simulink model "Project"  (R2017a)
settings: Solver=VariableStepAuto  StartTime=0.0  StopTime=20  FixedStep=0.01  RelTol=1e-3
values from neighbouring files (symbols this model uses):
  b = 2    [initial_condition_and_plots.m]
  c = 4    [initial_condition_and_plots.m]
  C = 2    [initial_condition_and_plots.m]
  Dmax = 3    [initial_condition_and_plots.m]
  init1 = [ -29 -27 pi/6]    [initial_condition_and_plots.m]
  init2 = [ -27 -24 2*pi/3]    [initial_condition_and_plots.m]
  init3 = [ -25 -21 pi/12]    [initial_condition_and_plots.m]
  init4 = [ -23 -19 pi/2]    [initial_condition_and_plots.m]
  init5 = [ -21 -12 5*pi/4]    [initial_condition_and_plots.m]
  K = 4    [initial_condition_and_plots.m]
  K_th = 3    [initial_condition_and_plots.m]
  Kij = 3    [initial_condition_and_plots.m]
  L = 20    [initial_condition_and_plots.m]
  r1k = 3    [initial_condition_and_plots.m]
  r2k = 4    [initial_condition_and_plots.m]
  x1k = 0    [initial_condition_and_plots.m]
  x2k = 15    [initial_condition_and_plots.m]
  y1k = -20    [initial_condition_and_plots.m]
  y2k = -5    [initial_condition_and_plots.m]
  yd = @(i) 4*i-20    [initial_condition_and_plots.m]
(part 2 of 2)

== system Project/Robot 4/Tracking Control ==
  note: u(6) =th _d
  note: u(5) = error_th
  note: u(4) = derror_y
  note: u(3) = error_y
  note: u(2) = derror_x
  note: u(1) = error_x
  X1 : Inport
  Xd : Inport  Port=2
  Y1 : Inport  Port=3
  Yd : Inport  Port=4
  TH1 : Inport  Port=5
  THc : Inport  Port=6
  Dc : Inport  Port=7
  CC : Inport  Port=8
  CCD : InportShadow  Port=8
  CCTH : InportShadow  Port=8
  Constant : Constant  Value=Dmax
  Derivative2 : Derivative
  Derivative3 : Derivative
  Fcn : Fcn  Expr=K*cos( u(5) )*u(7)
  Fcn1 : Fcn  Expr=K * cos(u(5)) * sin( u(5) + u(6) )*u(7)
  Fcn2 : Fcn  Expr=-K_th*u(5) +u(8)*( u(1)*u(4) - u(3)*u(2) )/( u(1)^2+u(3)^2 )
  Fcn3 : Fcn  Expr=atan2(-u(1),-u(2))
  Fcn4 : Fcn  Expr=(u(1)^2+u(2)^2)*(1/2)
  Fcn5 : Fcn  Expr=cos(u(5)+u(6))
  Integrator1 : Integrator  InitialCondition=init4(2)
  Integrator2 : Integrator  InitialCondition=init4(3)
  Integrator3 : Integrator  InitialCondition=init4(1)
  MinMax : MinMax  Inputs=2
  Mux : Mux  Inputs=8
  Mux1 : Mux  Inputs=2
  Mux2 : Mux  Inputs=2
  Product : Product
  Scope : Scope
  Sum : Sum  Inputs=|-+
  Sum1 : Sum  Inputs=|-+
  Sum2 : Sum  Inputs=|+-
  Sum3 : Sum  Inputs=|+-
  Sum4 : Sum  Inputs=|+-
  Switch : Switch  Criteria=u2 ~= 0
  Switch1 : Switch  Criteria=u2 ~= 0
  Unit Delay : UnitDelay  SampleTime=-1
  Unit Delay1 : UnitDelay  SampleTime=-1
  X : Outport
  Y : Outport  Port=2
  "TH " : Outport  Port=3
  V : Outport  Port=4
  "U " : Outport  Port=5
  wires:
  Integrator1/1 -> Y/1
  Integrator3/1 -> X/1
  Fcn2/1 -> "U "/1, Integrator2/1
  Fcn1/1 -> Sum3/1, Integrator1/1
  Product/1 -> Sum4/1, Integrator3/1
  Fcn5/1 -> Product/2
  Fcn/1 -> Product/1, V/1
  Constant/1 -> MinMax/1
  Integrator2/1 -> "TH "/1
  Mux/1 -> Fcn5/1, Fcn/1, Fcn2/1, Fcn1/1
  Mux1/1 -> Fcn3/1
  Derivative2/1 -> Sum4/2
  Sum2/1 -> Mux/5
  Yd/1 -> [yd], Sum1/1
  Mux2/1 -> Fcn4/1
  [error_y] -> Mux2/2
  Sum/1 -> Mux/1, [error_x]
  [dy1] -> Unit Delay1/1
  [error_x] -> Mux2/1
  Sum3/1 -> [dy1]
  X1/1 -> Sum/2
  TH1/1 -> Sum2/1
  [error_y] -> Mux1/1
  [yd] -> Derivative3/1
  Sum4/1 -> [dx1]
  Derivative3/1 -> Sum3/2
  [error_x] -> Mux1/2
  Sum1/1 -> Mux/3, [error_y]
  Y1/1 -> Sum1/2
  [xd] -> Derivative2/1
  MinMax/1 -> Scope/1, Mux/7
  Xd/1 -> Sum/1, [xd]
  CC/1 -> Mux/8
  Fcn4/1 -> Switch/1
  Dc/1 -> Switch/3
  CCD/1 -> Switch/2
  Switch/1 -> MinMax/2
  Fcn3/1 -> Switch1/1
  THc/1 -> Switch1/3
  Switch1/1 -> Sum2/2, Mux/6
  CCTH/1 -> Switch1/2
  [dx1] -> Unit Delay/1
  Unit Delay/1 -> Mux/2
  Unit Delay1/1 -> Mux/4

== system Project/Robot 5/Tracking Control ==
  note: u(1) = error_x
  note: u(2) = derror_x
  note: u(3) = error_y
  note: u(4) = derror_y
  note: u(5) = error_th
  note: u(6) =th _d
  X1 : Inport
  Xd : Inport  Port=2
  Y1 : Inport  Port=3
  Yd : Inport  Port=4
  TH1 : Inport  Port=5
  THc : Inport  Port=6
  Dc : Inport  Port=7
  CC : Inport  Port=8
  CCD : InportShadow  Port=8
  CCTH : InportShadow  Port=8
  Constant : Constant  Value=Dmax
  Derivative2 : Derivative
  Derivative3 : Derivative
  Fcn : Fcn  Expr=K*cos( u(5) )*u(7)
  Fcn1 : Fcn  Expr=K * cos(u(5)) * sin( u(5) + u(6) )*u(7)
  Fcn2 : Fcn  Expr=-K_th*u(5) +u(8)*( u(1)*u(4) - u(3)*u(2) )/( u(1)^2+u(3)^2 )
  Fcn3 : Fcn  Expr=atan2(-u(1),-u(2))
  Fcn4 : Fcn  Expr=(u(1)^2+u(2)^2)*(1/2)
  Fcn5 : Fcn  Expr=cos(u(5)+u(6))
  Integrator1 : Integrator  InitialCondition=init5(2)
  Integrator2 : Integrator  InitialCondition=init5(3)
  Integrator3 : Integrator  InitialCondition=init5(1)
  MinMax : MinMax  Inputs=2
  Mux : Mux  Inputs=8
  Mux1 : Mux  Inputs=2
  Mux2 : Mux  Inputs=2
  Product : Product
  Scope : Scope
  Sum : Sum  Inputs=|-+
  Sum1 : Sum  Inputs=|-+
  Sum2 : Sum  Inputs=|+-
  Sum3 : Sum  Inputs=|+-
  Sum4 : Sum  Inputs=|+-
  Switch : Switch  Criteria=u2 ~= 0
  Switch1 : Switch  Criteria=u2 ~= 0
  Unit Delay : UnitDelay  SampleTime=-1
  Unit Delay1 : UnitDelay  SampleTime=-1
  X : Outport
  Y : Outport  Port=2
  "TH " : Outport  Port=3
  V : Outport  Port=4
  "U " : Outport  Port=5
  wires:
  [dx1] -> Unit Delay/1
  CCTH/1 -> Switch1/2
  Switch1/1 -> Mux/6, Sum2/2
  THc/1 -> Switch1/3
  Fcn3/1 -> Switch1/1
  Switch/1 -> MinMax/2
  CCD/1 -> Switch/2
  Dc/1 -> Switch/3
  Fcn4/1 -> Switch/1
  CC/1 -> Mux/8
  Xd/1 -> [xd], Sum/1
  MinMax/1 -> Mux/7, Scope/1
  [xd] -> Derivative2/1
  Y1/1 -> Sum1/2
  Sum1/1 -> [error_y], Mux/3
  [error_x] -> Mux1/2
  Derivative3/1 -> Sum3/2
  Sum4/1 -> [dx1]
  [yd] -> Derivative3/1
  [error_y] -> Mux1/1
  TH1/1 -> Sum2/1
  X1/1 -> Sum/2
  Sum3/1 -> [dy1]
  [error_x] -> Mux2/1
  [dy1] -> Unit Delay1/1
  Sum/1 -> [error_x], Mux/1
  [error_y] -> Mux2/2
  Mux2/1 -> Fcn4/1
  Yd/1 -> Sum1/1, [yd]
  Sum2/1 -> Mux/5
  Derivative2/1 -> Sum4/2
  Mux1/1 -> Fcn3/1
  Mux/1 -> Fcn1/1, Fcn2/1, Fcn/1, Fcn5/1
  Integrator2/1 -> "TH "/1
  Constant/1 -> MinMax/1
  Fcn/1 -> V/1, Product/1
  Fcn5/1 -> Product/2
  Product/1 -> Integrator3/1, Sum4/1
  Fcn1/1 -> Integrator1/1, Sum3/1
  Fcn2/1 -> Integrator2/1, "U "/1
  Integrator3/1 -> X/1
  Integrator1/1 -> Y/1
  Unit Delay/1 -> Mux/2
  Unit Delay1/1 -> Mux/4

== system Project/THD1 /THD for obstacle 1 ==
  Constant : Constant  Value=yd(1)
  Constant1 : Constant  Value=-pi/2
  Constant2 : Constant  Value=pi/2
  Fcn : Fcn  Expr="u(1)  + atan2(u(2) - u(3) , u(4) - u(5))"
  Fcn1 : Fcn  Expr=atan2(u(1) , u(2))
  Mux : Mux  Inputs=5
  Mux1 : Mux  Inputs=2
  Sum : Sum  Inputs=|+++
  Sum1 : Sum  Inputs=|+-
  Sum2 : Sum  Inputs=|+-
  Switch : Switch  Criteria=u2 > Threshold  ZeroCross=off
  tag scope: g1a=global, thd1oa=global
  wires:
  [x1o1] -> Mux/4
  Fcn1/1 -> Sum/2
  Mux1/1 -> Fcn1/1
  [th1] -> Mux/1
  [x1] -> Mux/5
  [y1] -> Mux/3
  Mux/1 -> Fcn/1
  [y1o1] -> Mux/2
  Sum1/1 -> Mux1/1
  [x1] -> Sum2/2
  Fcn/1 -> [g1a], Sum/1
  Constant/1 -> Sum1/1
  Sum2/1 -> Mux1/2
  [g1a] -> Switch/2
  Sum/1 -> [thd1oa]
  Constant1/1 -> Switch/1
  Switch/1 -> Sum/3
  Constant2/1 -> Switch/3
  [y1] -> Sum1/2
  [Xd] -> Sum2/1

== system Project/THD1 /THD for obstacle 2 ==
  Constant : Constant  Value=yd(1)
  Constant1 : Constant  Value=-pi/2
  Constant2 : Constant  Value=pi/2
  Fcn : Fcn  Expr=u(1) + atan2(u(2) - u(3) , u(4) - u(5))
  Fcn1 : Fcn  Expr=atan2(u(1) , u(2))
  Mux : Mux  Inputs=5
  Mux1 : Mux  Inputs=2
  Sum : Sum  Inputs=|+++
  Sum1 : Sum  Inputs=|+-
  Sum2 : Sum  Inputs=|+-
  Switch : Switch  Criteria=u2 > Threshold  ZeroCross=off
  tag scope: g1b=global, thd1ob=global
  wires:
  [Xd] -> Sum2/1
  [y1] -> Sum1/2
  Constant2/1 -> Switch/3
  Switch/1 -> Sum/3
  Constant1/1 -> Switch/1
  Sum/1 -> [thd1ob]
  [g1b] -> Switch/2
  Sum2/1 -> Mux1/2
  Constant/1 -> Sum1/1
  Fcn/1 -> Sum/1, [g1b]
  [x1] -> Sum2/2
  Sum1/1 -> Mux1/1
  [y1o2] -> Mux/2
  Mux/1 -> Fcn/1
  [y1] -> Mux/3
  [x1] -> Mux/5
  [th1] -> Mux/1
  Mux1/1 -> Fcn1/1
  Fcn1/1 -> Sum/2
  [x1o2] -> Mux/4

== system Project/THD2/THD for obstacle 1 ==
  Constant : Constant  Value=yd(2)
  Constant1 : Constant  Value=-pi/2
  Constant2 : Constant  Value=pi/2
  Fcn : Fcn  Expr=u(1) + atan2(u(2) - u(3) , u(4) - u(5))
  Fcn1 : Fcn  Expr=atan2(u(1) , u(2))
  Mux : Mux  Inputs=5
  Mux1 : Mux  Inputs=2
  Sum : Sum  Inputs=|+++
  Sum1 : Sum  Inputs=|+-
  Sum2 : Sum  Inputs=|+-
  Switch : Switch  Criteria=u2 > Threshold  ZeroCross=off
  tag scope: g2a=global, thd2oa=global
  wires:
  [x2o1] -> Mux/4
  Fcn1/1 -> Sum/2
  Mux1/1 -> Fcn1/1
  [th2] -> Mux/1
  [x2] -> Mux/5
  [y2] -> Mux/3
  Mux/1 -> Fcn/1
  [y2o1] -> Mux/2
  Sum1/1 -> Mux1/1
  [x2] -> Sum2/2
  Fcn/1 -> [g2a], Sum/1
  Constant/1 -> Sum1/1
  Sum2/1 -> Mux1/2
  [g2a] -> Switch/2
  Sum/1 -> [thd2oa]
  Constant1/1 -> Switch/1
  Switch/1 -> Sum/3
  Constant2/1 -> Switch/3
  [y2] -> Sum1/2
  [Xd] -> Sum2/1

== system Project/THD2/THD for obstacle 2 ==
  Constant : Constant  Value=yd(2)
  Constant1 : Constant  Value=-pi/2
  Constant2 : Constant  Value=pi/2
  Fcn : Fcn  Expr=u(1)+ atan2(u(2) - u(3) , u(4) - u(5))
  Fcn1 : Fcn  Expr=atan2(u(1) , u(2))
  Mux : Mux  Inputs=5
  Mux1 : Mux  Inputs=2
  Sum : Sum  Inputs=|+++
  Sum1 : Sum  Inputs=|+-
  Sum2 : Sum  Inputs=|+-
  Switch : Switch  Criteria=u2 > Threshold  ZeroCross=off
  tag scope: g2b=global, thd2ob=global
  wires:
  [Xd] -> Sum2/1
  [y2] -> Sum1/2
  Constant2/1 -> Switch/3
  Switch/1 -> Sum/3
  Constant1/1 -> Switch/1
  Sum/1 -> [thd2ob]
  [g2b] -> Switch/2
  Sum2/1 -> Mux1/2
  Constant/1 -> Sum1/1
  Fcn/1 -> Sum/1, [g2b]
  [x2] -> Sum2/2
  Sum1/1 -> Mux1/1
  [y2o2] -> Mux/2
  Mux/1 -> Fcn/1
  [y2] -> Mux/3
  [x2] -> Mux/5
  [th2] -> Mux/1
  Mux1/1 -> Fcn1/1
  Fcn1/1 -> Sum/2
  [x2o2] -> Mux/4

== system Project/THD3/THD for obstacle 1 ==
  Constant : Constant  Value=yd(3)
  Constant1 : Constant  Value=-pi/2
  Constant2 : Constant  Value=pi/2
  Fcn : Fcn  Expr=atan2(u(3),u(5)) + atan2(u(2) - u(3) , u(4) - u(5))
  Fcn1 : Fcn  Expr=atan2(u(1) , u(2))
  Mux : Mux  Inputs=5
  Mux1 : Mux  Inputs=2
  Sum : Sum  Inputs=|+++
  Sum1 : Sum  Inputs=|+-
  Sum2 : Sum  Inputs=|+-
  Switch : Switch  Criteria=u2 > Threshold  ZeroCross=off
  tag scope: g3a=global, thd3oa=global
  wires:
  [x3o1] -> Mux/4
  Fcn1/1 -> Sum/2
  Mux1/1 -> Fcn1/1
  [th3] -> Mux/1
  [x3] -> Mux/5
  [y3] -> Mux/3
  Mux/1 -> Fcn/1
  [y3o1] -> Mux/2
  Sum1/1 -> Mux1/1
  [x3] -> Sum2/2
  Fcn/1 -> [g3a], Sum/1
  Constant/1 -> Sum1/1
  Sum2/1 -> Mux1/2
  [g3a] -> Switch/2
  Sum/1 -> [thd3oa]
  Constant1/1 -> Switch/1
  Switch/1 -> Sum/3
  Constant2/1 -> Switch/3
  [y3] -> Sum1/2
  [Xd] -> Sum2/1

== system Project/THD3/THD for obstacle 2 ==
  Constant : Constant  Value=yd(3)
  Constant1 : Constant  Value=-pi/2
  Constant2 : Constant  Value=pi/2
  Fcn : Fcn  Expr=atan2(u(3),u(5)) + atan2(u(2) - u(3) , u(4) - u(5))
  Fcn1 : Fcn  Expr=atan2(u(1) , u(2))
  Mux : Mux  Inputs=5
  Mux1 : Mux  Inputs=2
  Sum : Sum  Inputs=|+++
  Sum1 : Sum  Inputs=|+-
  Sum2 : Sum  Inputs=|+-
  Switch : Switch  Criteria=u2 > Threshold  ZeroCross=off
  tag scope: g3b=global, thd3ob=global
  wires:
  [Xd] -> Sum2/1
  [y3] -> Sum1/2
  Constant2/1 -> Switch/3
  Switch/1 -> Sum/3
  Constant1/1 -> Switch/1
  Sum/1 -> [thd3ob]
  [g3b] -> Switch/2
  Sum2/1 -> Mux1/2
  Constant/1 -> Sum1/1
  Fcn/1 -> Sum/1, [g3b]
  [x3] -> Sum2/2
  Sum1/1 -> Mux1/1
  [y3o2] -> Mux/2
  Mux/1 -> Fcn/1
  [y3] -> Mux/3
  [x3] -> Mux/5
  [th3] -> Mux/1
  Mux1/1 -> Fcn1/1
  Fcn1/1 -> Sum/2
  [x3o2] -> Mux/4

== system Project/THD4/THD for obstacle 1 ==
  Constant : Constant  Value=yd(4)
  Constant1 : Constant  Value=-pi/2
  Constant2 : Constant  Value=pi/2
  Fcn : Fcn  Expr=u(1)+ atan2(u(2) - u(3) , u(4) - u(5))
  Fcn1 : Fcn  Expr=atan2(u(1) , u(2))
  Mux : Mux  Inputs=5
  Mux1 : Mux  Inputs=2
  Sum : Sum  Inputs=|+++
  Sum1 : Sum  Inputs=|+-
  Sum2 : Sum  Inputs=|+-
  Switch : Switch  Criteria=u2 > Threshold  ZeroCross=off
  tag scope: g4a=global, thd4oa=global
  wires:
  [x4o1] -> Mux/4
  Fcn1/1 -> Sum/2
  Mux1/1 -> Fcn1/1
  [th4] -> Mux/1
  [x4] -> Mux/5
  [y4] -> Mux/3
  Mux/1 -> Fcn/1
  [y4o1] -> Mux/2
  Sum1/1 -> Mux1/1
  [x4] -> Sum2/2
  Fcn/1 -> [g4a], Sum/1
  Constant/1 -> Sum1/1
  Sum2/1 -> Mux1/2
  [g4a] -> Switch/2
  Sum/1 -> [thd4oa]
  Constant1/1 -> Switch/1
  Switch/1 -> Sum/3
  Constant2/1 -> Switch/3
  [y4] -> Sum1/2
  [Xd] -> Sum2/1

== system Project/THD4/THD for obstacle 2 ==
  Constant : Constant  Value=yd(4)
  Constant1 : Constant  Value=-pi/2
  Constant2 : Constant  Value=pi/2
  Fcn : Fcn  Expr=u(1) + atan2(u(2) - u(3) , u(4) - u(5))
  Fcn1 : Fcn  Expr=atan2(u(1) , u(2))
  Mux : Mux  Inputs=5
  Mux1 : Mux  Inputs=2
  Sum : Sum  Inputs=|+++
  Sum1 : Sum  Inputs=|+-
  Sum2 : Sum  Inputs=|+-
  Switch : Switch  Criteria=u2 > Threshold  ZeroCross=off
  tag scope: g4b=global, thd4ob=global
  wires:
  [Xd] -> Sum2/1
  [y4] -> Sum1/2
  Constant2/1 -> Switch/3
  Switch/1 -> Sum/3
  Constant1/1 -> Switch/1
  Sum/1 -> [thd4ob]
  [g4b] -> Switch/2
  Sum2/1 -> Mux1/2
  Constant/1 -> Sum1/1
  Fcn/1 -> Sum/1, [g4b]
  [x4] -> Sum2/2
  Sum1/1 -> Mux1/1
  [y4o2] -> Mux/2
  Mux/1 -> Fcn/1
  [y4] -> Mux/3
  [x4] -> Mux/5
  [th4] -> Mux/1
  Mux1/1 -> Fcn1/1
  Fcn1/1 -> Sum/2
  [x4o2] -> Mux/4

== system Project/THD5/THD for obstacle 1 ==
  Constant : Constant  Value=yd(5)
  Constant1 : Constant  Value=-pi/2
  Constant2 : Constant  Value=pi/2
  Fcn : Fcn  Expr=atan2(u(3),u(5)) + atan2(u(2) - u(3) , u(4) - u(5))
  Fcn1 : Fcn  Expr=atan2(u(1) , u(2))
  Mux : Mux  Inputs=5
  Mux1 : Mux  Inputs=2
  Sum : Sum  Inputs=|+++
  Sum1 : Sum  Inputs=|+-
  Sum2 : Sum  Inputs=|+-
  Switch : Switch  Criteria=u2 > Threshold  ZeroCross=off
  tag scope: g5a=global, thd5oa=global
  wires:
  [x5o1] -> Mux/4
  Fcn1/1 -> Sum/2
  Mux1/1 -> Fcn1/1
  [th5] -> Mux/1
  [x5] -> Mux/5
  [y5] -> Mux/3
  Mux/1 -> Fcn/1
  [y5o1] -> Mux/2
  Sum1/1 -> Mux1/1
  [x5] -> Sum2/2
  Fcn/1 -> [g5a], Sum/1
  Constant/1 -> Sum1/1
  Sum2/1 -> Mux1/2
  [g5a] -> Switch/2
  Sum/1 -> [thd5oa]
  Constant1/1 -> Switch/1
  Switch/1 -> Sum/3
  Constant2/1 -> Switch/3
  [y5] -> Sum1/2
  [Xd] -> Sum2/1

== system Project/THD5/THD for obstacle 2 ==
  Constant : Constant  Value=yd(5)
  Constant1 : Constant  Value=-pi/2
  Constant2 : Constant  Value=pi/2
  Fcn : Fcn  Expr=atan2(u(3),u(5)) + atan2(u(2) - u(3) , u(4) - u(5))
  Fcn1 : Fcn  Expr=atan2(u(1) , u(2))
  Mux : Mux  Inputs=5
  Mux1 : Mux  Inputs=2
  Sum : Sum  Inputs=|+++
  Sum1 : Sum  Inputs=|+-
  Sum2 : Sum  Inputs=|+-
  Switch : Switch  Criteria=u2 > Threshold  ZeroCross=off
  tag scope: g5b=global, thd5ob=global
  wires:
  [Xd] -> Sum2/1
  [y5] -> Sum1/2
  Constant2/1 -> Switch/3
  Switch/1 -> Sum/3
  Constant1/1 -> Switch/1
  Sum/1 -> [thd5ob]
  [g5b] -> Switch/2
  Sum2/1 -> Mux1/2
  Constant/1 -> Sum1/1
  Fcn/1 -> Sum/1, [g5b]
  [x5] -> Sum2/2
  Sum1/1 -> Mux1/1
  [y5o2] -> Mux/2
  Mux/1 -> Fcn/1
  [y5] -> Mux/3
  [x5] -> Mux/5
  [th5] -> Mux/1
  Mux1/1 -> Fcn1/1
  Fcn1/1 -> Sum/2
  [x5o2] -> Mux/4
